simulink model "Demonstration_of_P_I_PI_Controllers"  (R2022b)
settings: Solver=VariableStepAuto  StartTime=0.0  StopTime=20  MaxStep=1e-3  RelTol=1e-3
settings Model: Creator=Mo_7atem  LastModifiedBy=Mo_7atem

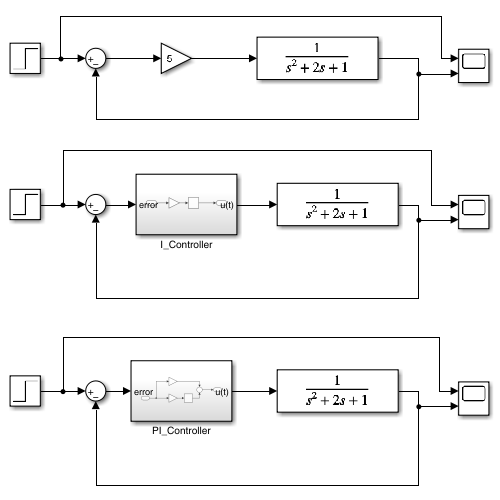
[thumbnail: Simulink's stored preview of the top-level diagram]
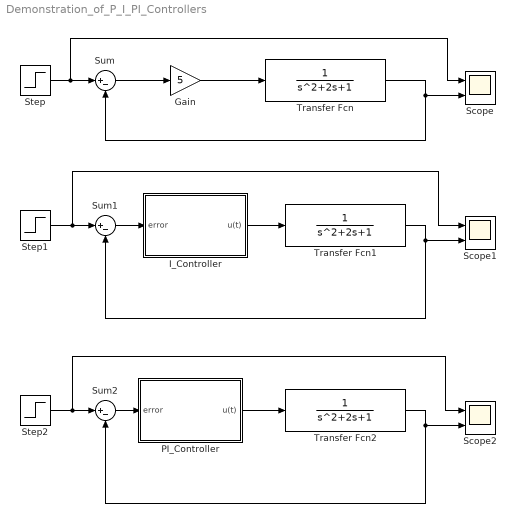
== system Demonstration_of_P_I_PI_Controllers ==
  Gain : Gain  Gain=5
  I_Controller : Subsystem
  PI_Controller : Subsystem
  Scope : Scope  NumInputPorts=2
  Scope1 : Scope  NumInputPorts=2
  Scope2 : Scope  NumInputPorts=2
  Step : Step  SampleTime=0
  Step1 : Step  SampleTime=0
  Step2 : Step  SampleTime=0
  Sum : Sum  Inputs=|+-
  Sum1 : Sum  Inputs=|+-
  Sum2 : Sum  Inputs=|+-
  Transfer Fcn : TransferFcn
  Transfer Fcn1 : TransferFcn
  Transfer Fcn2 : TransferFcn
  wires:
  Transfer Fcn/1 -> Sum/2, Scope/2
  Step/1 -> Scope/1, Sum/1
  Gain/1 -> Transfer Fcn/1
  Sum/1 -> Gain/1
  Transfer Fcn1/1 -> Sum1/2, Scope1/2
  Step1/1 -> Scope1/1, Sum1/1
  Sum1/1 -> I_Controller/1(error)
  I_Controller/1(u(t)) -> Transfer Fcn1/1
  PI_Controller/1(u(t)) -> Transfer Fcn2/1
  Sum2/1 -> PI_Controller/1(error)
  Step2/1 -> Sum2/1, Scope2/1
  Transfer Fcn2/1 -> Scope2/2, Sum2/2

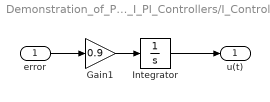
== system Demonstration_of_P_I_PI_Controllers/I_Controller ==
  error : Inport
  Gain1 : Gain  Gain=0.9
  Integrator : Integrator
  u(t) : Outport
  wires:
  Gain1/1 -> Integrator/1
  error/1 -> Gain1/1
  Integrator/1 -> u(t)/1

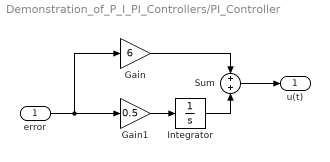
== system Demonstration_of_P_I_PI_Controllers/PI_Controller ==
  error : Inport
  Gain : Gain  Gain=6
  Gain1 : Gain  Gain=0.5
  Integrator : Integrator
  Sum : Sum
  u(t) : Outport
  wires:
  error/1 -> Gain/1, Gain1/1
  Gain1/1 -> Integrator/1
  Integrator/1 -> Sum/2
  Gain/1 -> Sum/1
  Sum/1 -> u(t)/1
